simulink model "slexDynamicSchedulingExample_org"  (Simulink 10.0)
settings: Solver=FixedStepAuto  StartTime=0.0  StopTime=1  FixedStep=1  RelTol=1e-3
libraries: simulink x2
settings Model: Creator=The MathWorks, Inc.  LastModifiedBy=bhisma
settings DataIOCC: ReturnWorkspaceOutputs=on
settings OptimizationCC: DefaultParameterBehavior=Inlined  PassReuseOutputArgsThreshold=0  LifeSpan=auto
settings DebuggingCC: UnderspecifiedInitializationDetection=Simplified  MergeDetectMultiDrivingBlocksExec=error  ParameterTunabilityLossMsg=error  SFUnexpectedBacktrackingDiag=error  SFNoUnconditionalDefaultTransitionDiag=error  SFExecutionAtInitializationDiag=warning
settings HardwareCC: ProdBitPerPointer=64  ProdBitPerSizeT=64  ProdBitPerPtrDiffT=64  ProdLargestAtomicFloat=Float  ProdIntDivRoundTo=Zero  ProdEndianess=LittleEndian  ProdWordSize=64  ProdHWDeviceType=Intel->x86-64 (Windows64)
settings ModelReferenceCC: PropagateSignalLabelsOutOfModel=on
settings SFSimCC: MATLABDynamicMemAlloc=off
settings RTWCC: GenerateReport=on  LaunchReport=on
settings CodeAppCC: ForceParamTrailComments=on  OperatorAnnotations=on  StateflowObjectComments=off
settings GRTTargetCC: TargetLangStandard=C99 (ISO)  CombineOutputUpdateFcns=on  GRTInterface=off
settings ConfigComp: CovMetricSettings=dwe  CovHtmlReporting=off  CovSaveCumulativeToWorkspaceVar=off  CovSaveSingleToWorkspaceVar=off

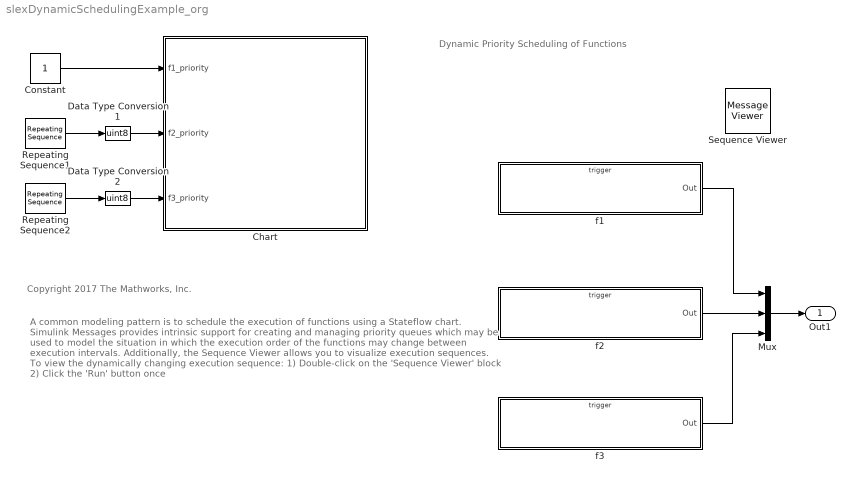
== system slexDynamicSchedulingExample_org ==
  note: A common modeling pattern is to schedule the execution of functions using a Stateflow chart. Simulink Messages provides intrinsic support for creating and managing priority queues which may be used to model the situation in which the execution order of the functions may change between execution intervals.
      |
      | Additionally, the Sequence Viewer allows you to visualize execution sequences. To view the dynamically changing execution sequence:
      | 1) Double-click on the 'Sequence Viewer' block
      | 2) Click the 'Run' button once
  note: Dynamic Priority Scheduling of Functions
  note: Copyright 2017 The Mathworks, Inc.
  Chart : Stateflow chart  TreatAsAtomicUnit=on
  Constant : Constant  OutDataTypeStr=uint8
  Data Type Conversion1 : DataTypeConversion  OutDataTypeStr=uint8
  Data Type Conversion2 : DataTypeConversion  OutDataTypeStr=uint8
  Mux : Mux  Inputs=3
  Repeating Sequence1 : simulink/Sources/Repeating Sequence  rep_seq_t=[0 1 2]  rep_seq_y=[2 3 2]
  Repeating Sequence2 : simulink/Sources/Repeating Sequence  rep_seq_t=[0 1 2]  rep_seq_y=[3 2 3]
  Sequence Viewer : MessageViewer  History=1000  WindowSettings=DataTag0
  f1 : Subsystem  TreatAsAtomicUnit=on
  f2 : Subsystem  TreatAsAtomicUnit=on
  f3 : Subsystem  TreatAsAtomicUnit=on
  Out1 : Outport  VectorParamsAs1DForOutWhenUnconnected=off
  wires:
  Repeating Sequence1/1 -> Data Type Conversion1/1
  Repeating Sequence2/1 -> Data Type Conversion2/1
  Constant/1 -> Chart/1(f1_priority)
  Data Type Conversion1/1 -> Chart/2(f2_priority)
  Data Type Conversion2/1 -> Chart/3(f3_priority)
  f1/1(Out) -> Mux/1
  f3/1(Out) -> Mux/3
  Mux/1 -> Out1/1
  f2/1(Out) -> Mux/2

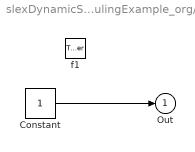
== system slexDynamicSchedulingExample_org/f1 ==
  f1 : TriggerPort  TriggerType=function-call  IsSimulinkFunction=on  FunctionName=f1  VariantControl=Variant
  Constant : Constant
  Out : Outport  VectorParamsAs1DForOutWhenUnconnected=off
  wires:
  Constant/1 -> Out/1

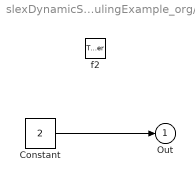
== system slexDynamicSchedulingExample_org/f2 ==
  f2 : TriggerPort  TriggerType=function-call  IsSimulinkFunction=on  FunctionName=f2  VariantControl=Variant
  Constant : Constant  Value=2
  Out : Outport  VectorParamsAs1DForOutWhenUnconnected=off
  wires:
  Constant/1 -> Out/1

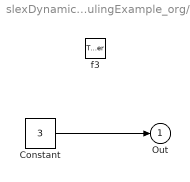
== system slexDynamicSchedulingExample_org/f3 ==
  f3 : TriggerPort  TriggerType=function-call  IsSimulinkFunction=on  FunctionName=f3  VariantControl=Variant
  Constant : Constant  Value=3
  Out : Outport  VectorParamsAs1DForOutWhenUnconnected=off
  wires:
  Constant/1 -> Out/1

== stateflow chart Chart ==
  settings: executeAtInitialization=1
  state fill_queue [parallel]
    settings: executionOrder=1
    note: To add a new function,
        | 1 - Create a new state here
        | 2 - Create a switch case within process function
    state f1 [parallel]
      du: request(1, f1_priority);
      settings: executionOrder=1
    state f2 [parallel]
      du: request(2, f2_priority);
      settings: executionOrder=2
    state f3 [parallel]
      du: request(3, f3_priority);
      settings: executionOrder=3
    state request(function_identifier, function_priority) [function]
      (default) -> (junction 13) : {
          |   pri = bitshift(function_priority, 5);
          |   queue.data = bitor(pri, function_identifier);
          |   send(queue);
          | }
  state process_queue [parallel]
    du: process();
    settings: executionOrder=2
    state process [function]
      (junction 16) -> (junction 15) [order 2]
      (default) -> (junction 16)
      (junction 17) -> (junction 16) : { discard(queue); }
      (junction 21) -> (junction 17)
      (junction 23) -> (junction 17)
      (junction 25) -> (junction 17)
      (junction 27) -> (junction 17)
      (junction 16) -> (junction 18) [order 1] : queue
      (junction 18) -> (junction 19) : {
          |    mask = uint8(bin2dec('11111'));
          |    function_id = bitand(queue.data, mask);
          | }
      (junction 19) -> (junction 20)
      (junction 20) -> (junction 21) [order 1] : [function_id == 1] {f1;}
      (junction 20) -> (junction 22) [order 2]
      (junction 22) -> (junction 23) [order 1] : [function_id == 2] {f2;}
      (junction 22) -> (junction 24) [order 2]
      (junction 24) -> (junction 25) [order 1] : [function_id == 3] {f3;}
      (junction 24) -> (junction 26) [order 2]
      (junction 26) -> (junction 27)
  data: function_identifier function_input uint8; function_priority function_input uint8; queue local double; f1_priority input uint8; f2_priority input uint8; f3_priority input uint8
